simulink model "MRAC_MCS_model"  (R2022a)
settings: Solver=VariableStepAuto  StartTime=0.0  StopTime=25  MaxStep=1e-3  RelTol=1e-3
InitFcn:
  | clear
  | clc
  | %% dati
  | %Plant
  | w0 = 5.278;
  | alfa1 = w0^2;
  | alfa3 = -1.402*w0^2;
  | alfa5 = 0.271*w0^2;
  | mu1 = 0.086;
  | mu3 = 0.1080;
  | %% MRAC MCS
  | % model reference
  | ta1 = 15;
  | zita = 0.62;
  | wn = -log(0.01)/(zita*ta1);
  | Am = [0 1; -wn^2 -2*zita*wn];
  | Bm = [0; wn^2];
  | Cm = eye(2);
  | Dm = [0; 0];
  | % control law
  | B = [0; 1];
  | Q = eye(2);
  | P = lyap(Am',Q);
  | C = P*B;
  | beta = 5;
  | alfa = 10*beta;
  | %disturbo
  | Ad = 0;
  | fd = 2;
  | %EMCS
  | gamma = 5;
  | epsilon = 0.01;
  | alfa1_hat = 0.8*w0^2;
settings Model: Creator=user  LastModifiedBy=user
settings SolverCC: ZeroCrossAlgorithm=Adaptive
settings DebuggingCC: IgnoredZcDiagnostic=none

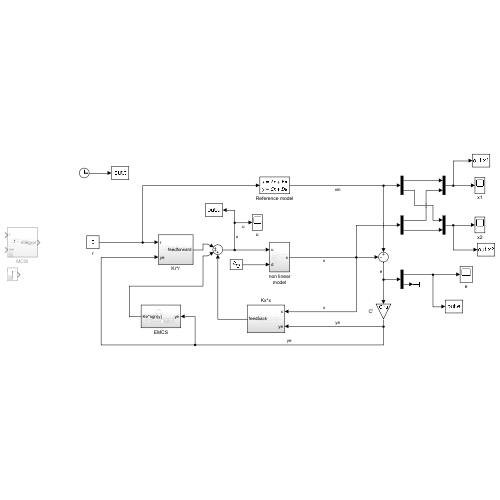
[thumbnail: Simulink's stored preview of the top-level diagram]
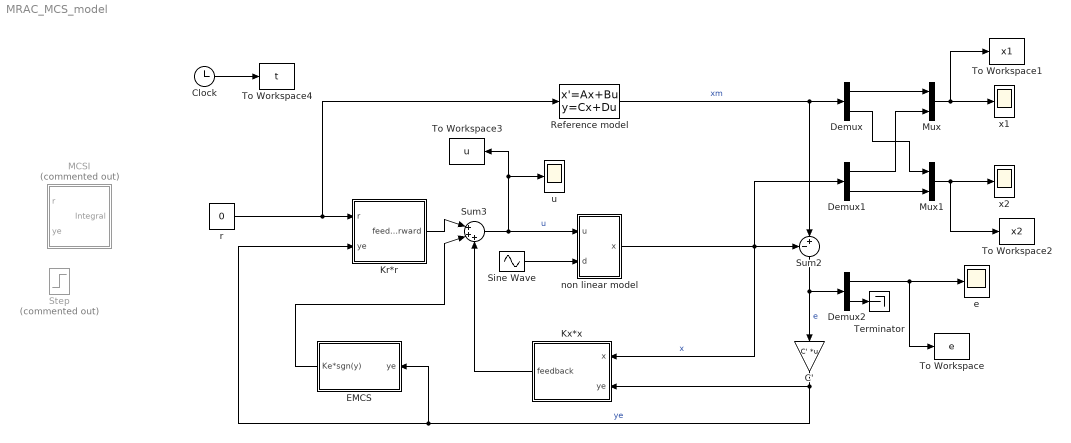
== system MRAC_MCS_model ==
  C' : Gain  Gain=C'  Multiplication=Matrix(K*u)
  Clock : Clock
  Demux : Demux  Outputs=2
  Demux1 : Demux  Outputs=2
  Demux2 : Demux  Outputs=2
  EMCS : Subsystem
  Kr*r : Subsystem
  Kx*x : Subsystem
  MCSI : Subsystem  Commented=on
  Mux : Mux  Inputs=2
  Mux1 : Mux  Inputs=2
  Reference model : StateSpace  A=Am  B=Bm  C=Cm  D=Dm  InitialCondition=[-1 -0.2]
  Sine Wave : Sin  Amplitude=Ad*0  Frequency=fd  SampleTime=0
  Step : Step  Commented=on  Time=15  After=5  SampleTime=0
  Sum2 : Sum  Inputs=-+|
  Sum3 : Sum  Inputs=|+++
  Terminator : Terminator
  To Workspace : ToWorkspace  VariableName=e  SampleTime=-1
      settings: Save2DSignal=2-D array (concatenate along first dimension)
  To Workspace1 : ToWorkspace  VariableName=x1  SampleTime=-1
      settings: Save2DSignal=2-D array (concatenate along first dimension)
  To Workspace2 : ToWorkspace  VariableName=x2  SampleTime=-1
      settings: Save2DSignal=2-D array (concatenate along first dimension)
  To Workspace3 : ToWorkspace  VariableName=u  SampleTime=-1
      settings: Save2DSignal=2-D array (concatenate along first dimension)
  To Workspace4 : ToWorkspace  VariableName=t  SampleTime=-1
      settings: Save2DSignal=2-D array (concatenate along first dimension)
  e : Scope
  non linear model : Subsystem
  r : Constant  Value=0
  u : Scope
  x1 : Scope
  x2 : Scope
  wires:
  Reference model/1 -> Demux/1, Sum2/2  "xm"
  r/1 -> Reference model/1, Kr*r/1(r)
  C'/1 -> Kr*r/2(ye), EMCS/1(ye), Kx*x/2(ye)  "ye"
  Sum2/1 -> Demux2/1, C'/1  "e"
  Sum3/1 -> non linear model/1(u), To Workspace3/1, u/1  "u"
  non linear model/1(x) -> Demux1/1, Sum2/1, Kx*x/1(x)  "x"
  Kr*r/1(feedforward) -> Sum3/1
  Demux2/1 -> To Workspace/1, e/1
  Demux2/2 -> Terminator/1
  Demux/1 -> Mux/1
  Demux1/1 -> Mux/2
  Demux/2 -> Mux1/1
  Demux1/2 -> Mux1/2
  Mux/1 -> To Workspace1/1, x1/1
  Mux1/1 -> To Workspace2/1, x2/1
  Clock/1 -> To Workspace4/1
  Sine Wave/1 -> non linear model/2(d)
  Kx*x/1(feedback) -> Sum3/3
  EMCS/1(Ke*sgn(y)) -> Sum3/2

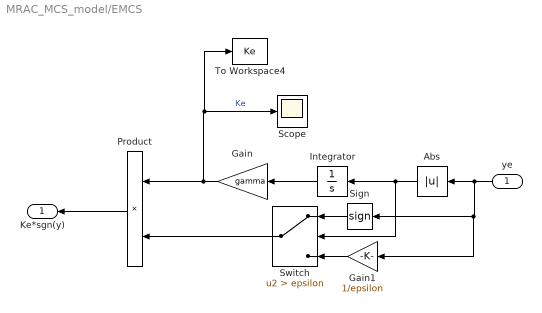
== system MRAC_MCS_model/EMCS ==
  ye : Inport
  Abs : Abs  SaturateOnIntegerOverflow=off
  Gain : Gain  Gain=gamma
  Gain1 : Gain  Gain=1/epsilon
  Integrator : Integrator
  Product : Product
  Scope : Scope
  Sign : Signum
  Switch : Switch  Criteria=u2 > Threshold  Threshold=epsilon  SaturateOnIntegerOverflow=off  InputSameDT=off
  To Workspace4 : ToWorkspace  VariableName=Ke  SampleTime=-1
      settings: Save2DSignal=2-D array (concatenate along first dimension)
  Ke*sgn(y) : Outport
  wires:
  Gain/1 -> To Workspace4/1, Scope/1, Product/1  "Ke"
  ye/1 -> Gain1/1, Sign/1, Abs/1
  Abs/1 -> Switch/2, Integrator/1
  Integrator/1 -> Gain/1
  Product/1 -> Ke*sgn(y)/1
  Gain1/1 -> Switch/3
  Sign/1 -> Switch/1
  Switch/1 -> Product/2

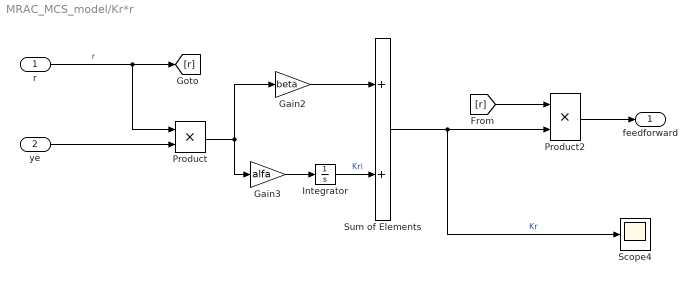
== system MRAC_MCS_model/Kr*r ==
  r : Inport
  ye : Inport  Port=2
  Gain2 : Gain  Gain=beta
  Gain3 : Gain  Gain=alfa
  Integrator : Integrator
  Product : Product
  Product2 : Product
  Scope4 : Scope
  Sum of Elements : Sum
  feedforward : Outport
  wires:
  r/1 -> [r], Product/1  "r"
  Gain3/1 -> Integrator/1
  ye/1 -> Product/2
  Product/1 -> Gain2/1, Gain3/1
  Integrator/1 -> Sum of Elements/2  "Kri"
  Sum of Elements/1 -> Scope4/1, Product2/2  "Kr"
  Gain2/1 -> Sum of Elements/1
  Product2/1 -> feedforward/1
  [r] -> Product2/1

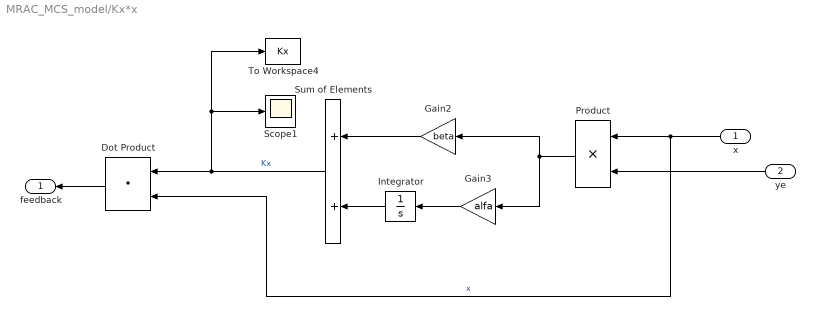
== system MRAC_MCS_model/Kx*x ==
  x : Inport
  ye : Inport  Port=2
  Dot Product : DotProduct  OutDataTypeStr=Inherit: Inherit via internal rule
  Gain2 : Gain  Gain=beta
  Gain3 : Gain  Gain=alfa
  Integrator : Integrator
  Product : Product
  Scope1 : Scope
  Sum of Elements : Sum
  To Workspace4 : ToWorkspace  VariableName=Kx  SampleTime=-1
      settings: Save2DSignal=2-D array (concatenate along first dimension)
  feedback : Outport
  wires:
  Dot Product/1 -> feedback/1
  x/1 -> Product/1, Dot Product/2  "x"
  Gain2/1 -> Sum of Elements/1
  Sum of Elements/1 -> Dot Product/1, To Workspace4/1, Scope1/1  "Kx"
  Product/1 -> Gain3/1, Gain2/1
  ye/1 -> Product/2
  Gain3/1 -> Integrator/1
  Integrator/1 -> Sum of Elements/2

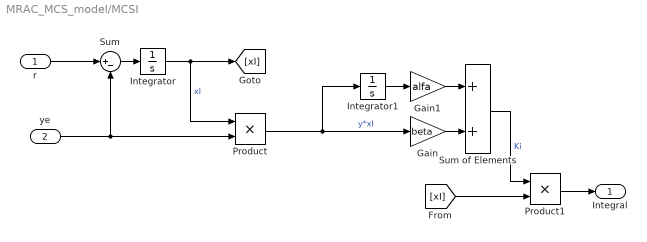
== system MRAC_MCS_model/MCSI ==
  r : Inport
  ye : Inport  Port=2
  Gain : Gain  Gain=beta
  Gain1 : Gain  Gain=alfa
  Integrator : Integrator
  Integrator1 : Integrator
  Product : Product
  Product1 : Product
  Sum : Sum  Inputs=|+-
  Sum of Elements : Sum
  Integral : Outport
  wires:
  Sum/1 -> Integrator/1
  Integrator/1 -> [xI], Product/1  "xI"
  ye/1 -> Product/2, Sum/2
  r/1 -> Sum/1
  Product/1 -> Integrator1/1, Gain/1  "y*xI"
  Integrator1/1 -> Gain1/1
  Gain/1 -> Sum of Elements/2
  Gain1/1 -> Sum of Elements/1
  Product1/1 -> Integral/1
  Sum of Elements/1 -> Product1/1  "Ki"
  [xI] -> Product1/2

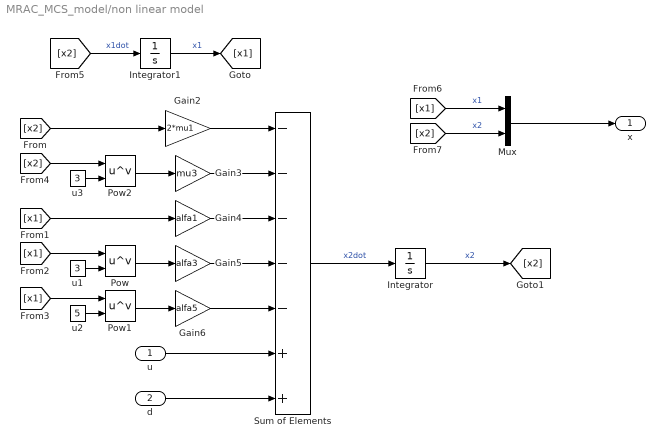
== system MRAC_MCS_model/non linear model ==
  u : Inport
  d : Inport  Port=2
  Gain2 : Gain  Gain=2*mu1
  Gain3 : Gain  Gain=mu3
  Gain4 : Gain  Gain=alfa1
  Gain5 : Gain  Gain=alfa3
  Gain6 : Gain  Gain=alfa5
  Integrator : Integrator  InitialCondition=-0.18
  Integrator1 : Integrator  InitialCondition=-1.2
  Mux : Mux  Inputs=2
  Pow : Math  Operator=pow  RndMeth=Zero
  Pow1 : Math  Operator=pow  RndMeth=Zero
  Pow2 : Math  Operator=pow  RndMeth=Zero
  Sum of Elements : Sum  Inputs=-----++
  u1 : Constant  Value=3
  u2 : Constant  Value=5
  u3 : Constant  Value=3
  x : Outport
  wires:
  [x2] -> Gain2/1
  [x1] -> Mux/1  "x1"
  [x1] -> Pow1/1
  [x2] -> Pow2/1
  Integrator/1 -> [x2]  "x2"
  Pow1/1 -> Gain6/1
  Pow2/1 -> Gain3/1
  Mux/1 -> x/1
  u3/1 -> Pow2/2
  Sum of Elements/1 -> Integrator/1  "x2dot"
  [x1] -> Gain4/1
  u/1 -> Sum of Elements/6
  u2/1 -> Pow1/2
  Pow/1 -> Gain5/1
  Gain2/1 -> Sum of Elements/1
  u1/1 -> Pow/2
  Integrator1/1 -> [x1]  "x1"
  [x2] -> Integrator1/1  "x1dot"
  [x1] -> Pow/1
  Gain4/1 -> Sum of Elements/3
  Gain3/1 -> Sum of Elements/2
  Gain5/1 -> Sum of Elements/4
  Gain6/1 -> Sum of Elements/5
  [x2] -> Mux/2  "x2"
  d/1 -> Sum of Elements/7
